simulink model "simulink_main"  (R2021b)
settings: Solver=ode23tb  StartTime=0.0  StopTime=1260  RelTol=1e-4
libraries: spsFourierLib x2, spsThreePhaseProgrammableVoltageSourceLib x1, spsSimplifiedSynchronousMachinepuUnitsLib x1, spsGroundLib x1, spspowerguiLib x1
settings Model: Creator=The MathWorks, Inc.  LastModifiedBy=ARUN SHARMA
settings SolverCC: ZeroCrossAlgorithm=Adaptive  AlgebraicLoopSolver=TrustRegion
settings DataIOCC: SaveFormat=Array  ReturnWorkspaceOutputs=off  SignalLoggingName=sigsOut
settings OptimizationCC: BlockReduction=off  BooleanDataType=off  ExpressionDepthLimit=2147483647  InitFltsAndDblsToZero=on  EfficientMapNaN2IntZero=off  LifeSpan=inf
settings DebuggingCC: UnderspecifiedInitializationDetection=Classic  MergeDetectMultiDrivingBlocksExec=none  CheckExecutionContextPreStartOutputMsg=on  SignalResolutionControl=TryResolveAllWithWarning  IgnoredZcDiagnostic=none  MultiTaskDSMMsg=warning  MultiTaskCondExecSysMsg=none  SigSpecEnsureSampleTimeMsg=none  IntegerOverflowMsg=none  FcnCallInpInsideContextMsg=warning  StateNameClashWarn=warning  SFUnexpectedBacktrackingDiag=warning  SFNoUnconditionalDefaultTransitionDiag=warning  SFExecutionAtInitializationDiag=none  SFMachineParentedDataDiag=warning  IntegerSaturationMsg=none  ArithmeticOperatorsInVariantConditions=warning
settings HardwareCC: ProdBitPerPointer=32  ProdBitPerSizeT=32  ProdBitPerPtrDiffT=32  ProdLargestAtomicFloat=None  ProdIntDivRoundTo=Undefined  ProdEndianess=Unspecified  ProdWordSize=32  ProdHWDeviceType=32-bit Generic  TargetUnknown=on
settings ModelReferenceCC: PropagateSignalLabelsOutOfModel=off
settings SFSimCC: SimUseLocalCustomCode=off  CustomCodeUndefinedFunction=UseInterfaceOnly
settings RTWCC: RTWUseLocalCustomCode=off
settings CodeAppCC: StateflowObjectComments=on
settings GRTTargetCC: TargetLangStandard=C89/C90 (ANSI)  CombineOutputUpdateFcns=off  GRTInterface=on
settings ConfigComp: CovMetricSettings=dw  CovSaveCumulativeToWorkspaceVar=on  CovSaveSingleToWorkspaceVar=on  CovExternalEMLEnable=off  CovSFcnEnable=off
settings SimscapeCC: SimscapeNormalizeSystem=off

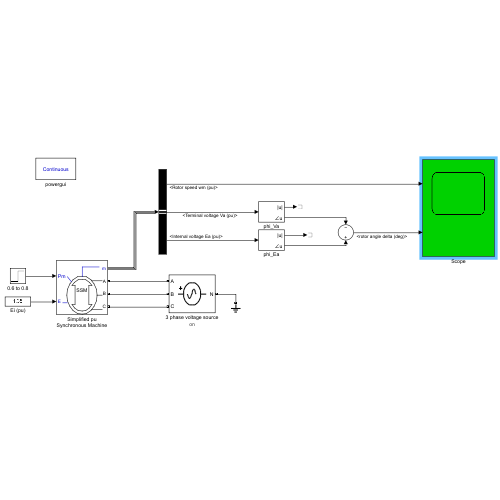
[thumbnail: Simulink's stored preview of the top-level diagram]
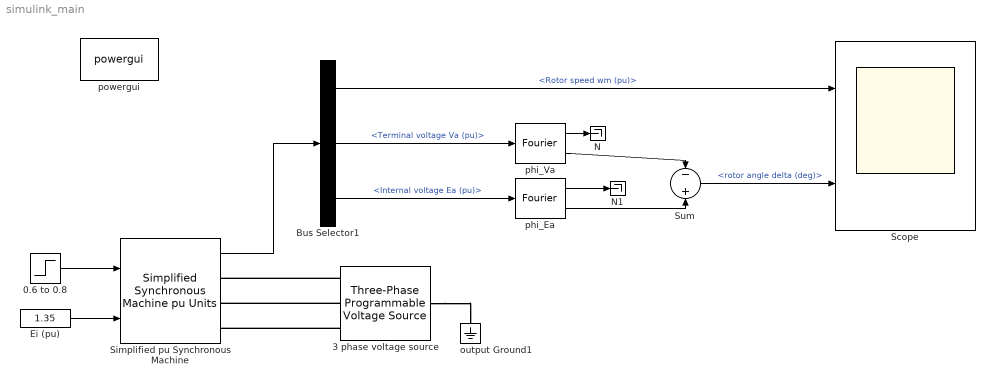
== system simulink_main ==
  0.6 to 0.8 : Step  Time=2  Before=0.6  After=0.8  SampleTime=0
  3 phase voltage source : spsThreePhaseProgrammableVoltageSourceLib/Three-Phase Programmable Voltage Source  PositiveSequence="[13.8e3 0  60]"  VariationEntity=None  VariationType=Step  VariationTypeAlt=Step  VariationStep=-0.5  VariationRate=10  VariationMagnitude=0.3  VariationFrequency=2  VariationTiming=[0.1 1.2]  VariationPhaseA=off  Amplitudes=[1 0.8 1.2 1.0]  TimeValues=[0 0.1 0.15 0.2]  HarmonicGeneration=off  HarmonicA=[3 0.2 -25 0]  HarmonicB="[2 0.15  35 2]"  Timing="[0.05  3]"  BusType=swing  Pref=-120e6  Qref=-160e6  Qmin=-inf  Qmax=inf
      settings: AttributesFormatString=%<Mask>
  Bus Selector1 : BusSelector  OutputSignals=Rotor speed wm (pu),Terminal voltage Va (pu),Internal voltage Ea (pu)
  Ei (pu) : Constant  Value=1.35
  N : Terminator
  N1 : Terminator
  Scope : Scope  NumInputPorts=2
  Simplified pu Synchronous Machine : spsSimplifiedSynchronousMachinepuUnitsLib/Simplified Synchronous Machine pu Units  ConnectionType=3-wire Y  MechanicalLoad=Mechanical power Pm  MeasurementBus=off  NominalParameters="[  100e6, 13800, 60 ]"  Mechanical="[ 9.94,  0.138, 1 ]"  InternalRL="[ 0  0.65 ]"  InitialConditions=[0 16.79 0.75 0.75 0.75 -36.87 -156.87 83.13]  IterativeDiscreteModel=Trapezoidal non iterative  TsBlock=-1  TsPowergui=0  LoadFlowParameters=[2 0 0 0]  Units=0  BusType=swing  Pref=0.6  Qref=0  Qmin=-Inf  Qmax=Inf  PLF=0  QLF=0
      settings: AttributesFormatString=\n  SourceProductBaseCode=PS
  Sum : Sum  Inputs=-+  InputSameDT=on  SaturateOnIntegerOverflow=on  OutDataTypeStr=Inherit: Same as first input
  output Ground1 : spsGroundLib/Ground  LConnTagsString=a
  phi_Ea : spsFourierLib/Fourier  Freq=60  n=1  InInit=[0, 0]  Ts=0
      settings: SourceProductBaseCode=PS
  phi_Va : spsFourierLib/Fourier  Freq=60  n=1  InInit=[0, 0]  Ts=0
      settings: SourceProductBaseCode=PS
  powergui : spspowerguiLib/powergui  Priority=2  SimulationMode=Continuous  SampleTime=0  frequency=60  Iterations=50  frequencyindice=60  Pbase=1e6  ErrMax=0.0001  UnitsV=V  UnitsW=kW  buscounter=0  FunctionMessages=off  echomessages=off  EnableUseOfTLC=off  CurrentSourceSwitches=off  DisableSnubberDevices=on  DisableRonSwitches=off  DisableVfSwitches=off  DisplayEquations=off  AutomaticDiscreteSolvers=off  SolverType=Tustin  Interpol=off  ExternalGateDelay=off  methode=off  Ts=0  x0status=blocks  SPID=on  SwTol=0  HookPort=off  NonlinearTolerance=1e-4  nMaxIteration=100  ContinueOnMaxIteration=off  RestoreLinks=warning  ResistiveCurrentMeasurement=off  Frange=[0:2:500]  Ylog=off  Xlog=on  ShowGrid=off  save=off  variable=ZData  structure=0  ZoomFFT=on  StartTime=0.0  cycles=1  DisplayStyle=off  fundamental=60  FreqAxis=off  MaxFrequency=1000  frequencyindicesteady=1  RmsSteady=1  display=off
  wires:
  Simplified pu Synchronous Machine/1 -> Bus Selector1/1
  Ei (pu)/1 -> Simplified pu Synchronous Machine/2
  Bus Selector1/1 -> Scope/1  "<Rotor speed wm (pu)>"
  0.6 to 0.8/1 -> Simplified pu Synchronous Machine/1
  phi_Va/2 -> Sum/1
  Bus Selector1/3 -> phi_Ea/1  "<Internal voltage Ea (pu)>"
  phi_Va/1 -> N/1
  Bus Selector1/2 -> phi_Va/1  "<Terminal voltage Va (pu)>"
  phi_Ea/2 -> Sum/2
  phi_Ea/1 -> N1/1
  Sum/1 -> Scope/2  "<rotor angle delta (deg)>"
  connections:
  3 phase voltage source/LConn1 -- output Ground1/LConn1
  3 phase voltage source/RConn1 -- Simplified pu Synchronous Machine/RConn1
  3 phase voltage source/RConn2 -- Simplified pu Synchronous Machine/RConn2
  3 phase voltage source/RConn3 -- Simplified pu Synchronous Machine/RConn3
